simulink model "controlScheme_rt"  (R2017a)
settings: Solver=ode4  StartTime=0.0  StopTime=5000  FixedStep=1/30  RelTol=1e-3  EnableMultiTasking=on
PreLoadFcn:
  | target_ip_addr = '192.168.1.5';
  | target_user = 'root';
model workspace (MAT data in the model file):
  N_obj = Simulink.Parameter
  N_obj.Value = 1
  N_obj.DataType = 'auto'
  N_obj.Min = 0
  N_obj.Max = 4
  N_obj.Dimensions = [1 1]
  target_ip_addr = '147.32.86.138'
undefined symbols (not defined in the file): H, H_R
libraries: TB_blk_library x2
settings Model: SimulationMode=external  ExtModeTrigDuration=200000  Creator=krecmich  LastModifiedBy=gurtnmar
settings DataIOCC: LimitDataPoints=on  SaveFormat=Array
settings OptimizationCC: ExpressionDepthLimit=2147483647  LifeSpan=1
settings DebuggingCC: UnderspecifiedInitializationDetection=Classic  MergeDetectMultiDrivingBlocksExec=none  SolverPrmCheckMsg=warning  StateNameClashWarn=warning  SFUnexpectedBacktrackingDiag=warning  SFNoUnconditionalDefaultTransitionDiag=warning  SFExecutionAtInitializationDiag=none
settings HardwareCC: ProdBitPerLong=64  ProdLargestAtomicFloat=None  ProdHWDeviceType=Intel->x86-64
settings ModelReferenceCC: PropagateSignalLabelsOutOfModel=off
settings SFSimCC: MATLABDynamicMemAlloc=off
settings RTWCC: SystemTargetFile=ert_linux.tlc  MakeCommand="make_rtw OPT_OPTS=\"-O2 -ggdb -Wall\" CC=aarch64-linux-gnu-gcc CPP=aarch64-linux-gnu-gcc"  TemplateMakefile=ert_linux.tmf  Description=Linux Embedded Coder
settings CodeAppCC: IgnoreCustomStorageClasses=off  CustomSymbolStrType=$N$R$M  InternalIdentifier=Classic
settings STFCustomTargetCC: TargetLangStandard=C99 (ISO)  ModelReferenceCompliant=off  CombineOutputUpdateFcns=on  ERTCustomFileBanners=on  RemoveResetFunc=on  MATLABClassNameForMDSCustomization=Simulink.SoftwareTarget.ERTCustomization  GRTInterface=off  SystemTargetFile=ert_linux.tlc
settings ERTTargetCC: TargetLangStandard=C99 (ISO)  MultiwordLength=2048  ModelReferenceCompliant=off  ParMdlRefBuildCompliant=off  CompOptLevelCompliant=off  ConcurrentExecutionCompliant=off  ERTFirstTimeCompliant=off  SupportContinuousTime=on  SupportNonInlinedSFcns=on  ModelStepFunctionPrototypeControlCompliant=off  CPPClassGenCompliant=off  UseToolchainInfoCompliant=off  ExtMode=on  ExtModeMexArgs='147.32.86.138'  ERTCustomFileTemplate=ert_linux_file_process.tlc  ConvertIfToSwitch=off  SuppressUnreachableDefaultCases=off
settings ConfigComp: CovMetricSettings=dw  CovHtmlReporting=on  CovSaveCumulativeToWorkspaceVar=on  CovSaveSingleToWorkspaceVar=on  CovExternalEMLEnable=off

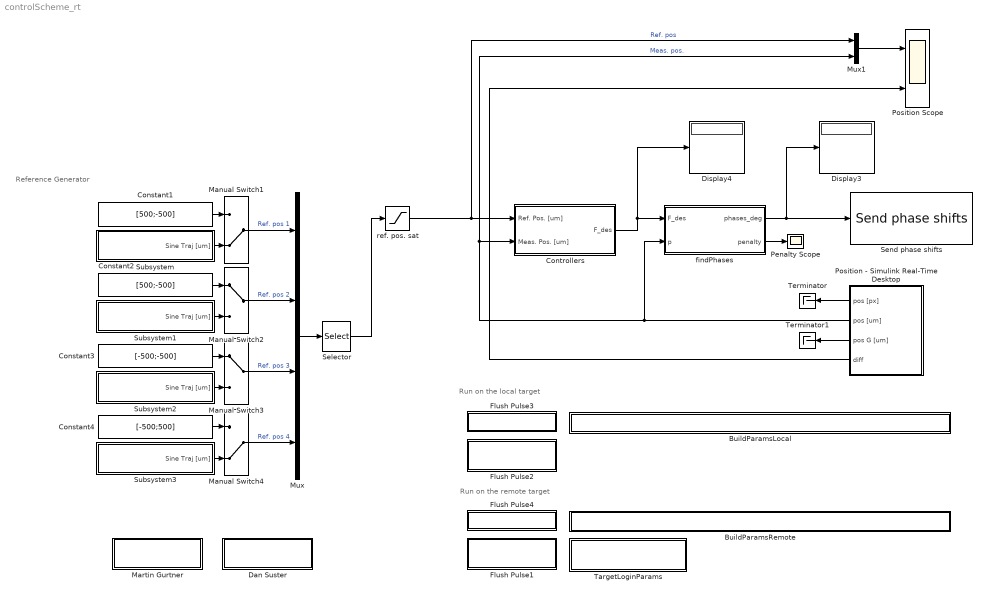
== system controlScheme_rt ==
  note: Reference Generator
  note: Run on the remote target
  note: Run on the local target
  BuildParamsLocal : Subsystem  mask{make_command='make_rtw OPT_OPTS="-O2 -ggdb -Wall" CC=gcc'}
      mask prompts: make_command "MakeCommand"
      mask Display: disp(get_param(gcb, 'make_command'));
  BuildParamsRemote : Subsystem  mask{make_command='make_rtw OPT_OPTS="-O2 -ggdb -Wall" CC=aarch64-linux-gnu-gcc CPP=aarch64-linux-gnu-gcc'}
      mask prompts: make_command "MakeCommand"
      mask Display: disp(get_param(gcb, 'make_command'));
  Constant1 : Constant  Value=[500;-500]
  Constant2 : Constant  Value=[500;-500]
  Constant3 : Constant  Value=[-500;-500]
  Constant4 : Constant  Value=[-500;500]
  Controllers : Subsystem  mask{P_const=300e-14, F_max=30e-11}
      mask prompts: P_const "P constant"; F_max "F max"
  Dan Suster : Subsystem
      settings: OpenFcn=|
      | wrkspc = get_param('controlScheme_rt', 'modelworkspace')
      | N_obj_sp = getVariable(wrkspc, 'N_obj')
      | N_obj = N_obj_sp.Value;
      | ip_addr = getVariable(wrkspc, 'target_ip_addr');
      | 
      | tb = twinbeam(ip_addr, 30000)
      | img_G = tb.get('backpropagated');
      | img_R = tb.get('backpropagated_r');
      | delete(tb);
      | %%
      | fig = figure(25);
      | imshow(img_G);
      | [x, y] = ginput(N_obj);
      | positions = [y, x];
      | positions_G = [positions(:,2)'; positions(:,1)'];
      | 
      | imshow(img_R);
      | [x, y] = ginput(N_obj);
      | positions = [y, x];
      | positions_R = [positions(:,2)'; positions(:,1)'];
      | 
      | close(fig);
      | %%
      | message = [uint8('t'), uint8('i'), typecast(uint16(numel(positions_G)/2),'uint8'), typecast(uint16(numel(positions_R)/2),'uint8'), typecast(uint16(positions_G(:)'),'uint8'), typecast(uint16(positions_R(:)'),'uint8')];
      | %%
      | conn = tcpclient('147.32.86.138', 30003, 'ConnectTimeout', 5);
      | write(conn, message);
      | clear conn;
      mask Display: disp('(Re)Initialize\ntracker')
  Display3 : Display
  Display4 : Display
  Flush Pulse1 : Subsystem
      settings: OpenFcn=|
      | % get the login credentials from the TargetLoginParams block
      | trgt_ip = eval(get_param(strcat(gcs, '/TargetLoginParams'), 'trgt_ip_addr'));
      | trgt_user = eval(get_param(strcat(gcs, '/TargetLoginParams'), 'trgt_username'));
      | 
      | % Set the IP address of the target
      | set_param(getActiveConfigSet(gcs), 'ExtModeMexArgs', sprintf('''%s''', trgt_ip));
      | 
      | system(['./run_model.sh ', get_param(bdroot(gcbh),'name'),' ',trgt_ip,' ',trgt_user]);
      mask Display: disp('Deploy and\nwait for connection')
  Flush Pulse2 : Subsystem
      settings: OpenFcn=|
      | configSet = getActiveConfigSet(gcs);
      | % Set the make command params
      | set_param( configSet, 'MakeCommand', '''make_rtw OPT_OPTS="-O2 -ggdb -Wall" CC=gcc''')
      | 
      | % Set the IP address of the target to the localhost
      | set_param(getActiveConfigSet(gcs), 'ExtModeMexArgs', '''127.0.0.1''')
      | 
      | system(['./run_model.sh ', get_param(bdroot(gcbh),'name')]);
      mask Display: disp('Deploy and\nwait for connection')
  Flush Pulse3 : Subsystem
      settings: OpenFcn=|
      | configSet = getActiveConfigSet(gcs);
      | % Set the make command params
      | set_param( configSet, 'MakeCommand', eval(get_param(strcat(gcs, '/BuildParamsLocal'), 'make_command')))
      | 
      | % Build the model
      | rtwbuild(gcs);
      mask Display: disp('Build')
  Flush Pulse4 : Subsystem
      settings: OpenFcn=|
      | configSet = getActiveConfigSet(gcs);
      | % Set the make command params
      | set_param( configSet, 'MakeCommand', eval(get_param(strcat(gcs, '/BuildParamsRemote'), 'make_command')))
      | 
      | % Build the model
      | rtwbuild(gcs);
      mask Display: disp('Build')
  Manual Switch1 : ManualSwitch  CurrentSetting=0
  Manual Switch2 : ManualSwitch
  Manual Switch3 : ManualSwitch
  Manual Switch4 : ManualSwitch  CurrentSetting=0
  Martin Gurtner : Subsystem
      settings: OpenFcn=|
      | wrkspc = get_param('controlScheme_rt', 'modelworkspace')
      | N_obj_sp = getVariable(wrkspc, 'N_obj')
      | N_obj = N_obj_sp.Value;
      | ip_addr = getVariable(wrkspc, 'target_ip_addr');
      | 
      | tb = twinbeam(ip_addr, 30000)
      | tb.tracker_init(N_obj);
      | clear conn;
      | delete(tb);
      mask Display: disp('(Re)Initialize\ntracker')
  Mux : Mux
  Mux1 : Mux  Inputs=2
  Penalty Scope : Scope
  Position - Simulink Real-Time Desktop : Subsystem  VariantControl=(default)
  Position Scope : Scope  NumInputPorts=2
  Selector : Selector  InputPortWidth=8  IndexOptions=Index vector (dialog)  Indices=[1:2*N_obj]  OutputSizes=1
  Send phase shifts : TB_blk_library/Send phase shifts  Ts=1/30  ip_addr=target_ip_addr  tcp_port=30001
  Subsystem : Subsystem  mask{xAmpl=400, xFreq=2*pi/50, xOff=0, yAmpl=400, yFreq=2*pi/50, yOff=pi/2}
      mask prompts: xAmpl "Amplitude"; xFreq "Frequency"; xOff "Phase Offset"; yAmpl "Amplitude"; yFreq "Frequency"; yOff "Phase Offset"
      mask DialogControl Container3 Prompt: Sine Trajectory Generator
      mask Display:
      | xAmpl = get_param(gcb, 'xAmpl');
      | xFreq = get_param(gcb, 'xFreq');
      | xOff = get_param(gcb, 'xOff');
      | yAmpl = get_param(gcb, 'yAmpl');
      | yFreq = get_param(gcb, 'yFreq');
      | yOff = get_param(gcb, 'yOff');
      | 
      | fprintf('x:%s sin(%s*t + %s)\ny:%s sin(%s*t + %s)', xAmpl, xFreq, xOff, yAmpl, yFreq, yOff)
  Subsystem1 : Subsystem  mask{xAmpl=300, xFreq=2*pi/40, xOff=pi/2, yAmpl=300, yFreq=2*pi/40, yOff=pi}
      mask prompts: xAmpl "Amplitude"; xFreq "Frequency"; xOff "Phase Offset"; yAmpl "Amplitude"; yFreq "Frequency"; yOff "Phase Offset"
      mask DialogControl Container3 Prompt: Sine Trajectory Generator
      mask Display:
      | xAmpl = get_param(gcb, 'xAmpl');
      | xFreq = get_param(gcb, 'xFreq');
      | xOff = get_param(gcb, 'xOff');
      | yAmpl = get_param(gcb, 'yAmpl');
      | yFreq = get_param(gcb, 'yFreq');
      | yOff = get_param(gcb, 'yOff');
      | 
      | fprintf('x:%s sin(%s*t + %s)\ny:%s sin(%s*t + %s)', xAmpl, xFreq, xOff, yAmpl, yFreq, yOff)
  Subsystem2 : Subsystem  mask{xAmpl=400, xFreq=2*pi/40, xOff=pi, yAmpl=400, yFreq=2*pi/40, yOff=3*pi/2}
      mask prompts: xAmpl "Amplitude"; xFreq "Frequency"; xOff "Phase Offset"; yAmpl "Amplitude"; yFreq "Frequency"; yOff "Phase Offset"
      mask DialogControl Container3 Prompt: Sine Trajectory Generator
      mask Display:
      | xAmpl = get_param(gcb, 'xAmpl');
      | xFreq = get_param(gcb, 'xFreq');
      | xOff = get_param(gcb, 'xOff');
      | yAmpl = get_param(gcb, 'yAmpl');
      | yFreq = get_param(gcb, 'yFreq');
      | yOff = get_param(gcb, 'yOff');
      | 
      | fprintf('x:%s sin(%s*t + %s)\ny:%s sin(%s*t + %s)', xAmpl, xFreq, xOff, yAmpl, yFreq, yOff)
  Subsystem3 : Subsystem  mask{xAmpl=400, xFreq=2*pi/40, xOff=3*pi/2, yAmpl=400, yFreq=2*pi/40, yOff=2*pi}
      mask prompts: xAmpl "Amplitude"; xFreq "Frequency"; xOff "Phase Offset"; yAmpl "Amplitude"; yFreq "Frequency"; yOff "Phase Offset"
      mask DialogControl Container3 Prompt: Sine Trajectory Generator
      mask Display:
      | xAmpl = get_param(gcb, 'xAmpl');
      | xFreq = get_param(gcb, 'xFreq');
      | xOff = get_param(gcb, 'xOff');
      | yAmpl = get_param(gcb, 'yAmpl');
      | yFreq = get_param(gcb, 'yFreq');
      | yOff = get_param(gcb, 'yOff');
      | 
      | fprintf('x:%s sin(%s*t + %s)\ny:%s sin(%s*t + %s)', xAmpl, xFreq, xOff, yAmpl, yFreq, yOff)
  TargetLoginParams : Subsystem  mask{trgt_ip_addr='147.32.86.138', trgt_username='nvidia'}
      mask prompts: trgt_ip_addr "Target IP address"; trgt_username "Target username"
      mask Display:
      | ip_addr = get_param(gcb, 'trgt_ip_addr');
      | user = get_param(gcb, 'trgt_username');
      | 
      | fprintf('IP addr:\t %s\n User:\t %s ', ip_addr, user);
  Terminator : Terminator
  Terminator1 : Terminator
  findPhases : MATLAB Function  TreatAsAtomicUnit=on
  ref. pos. sat : Saturate  UpperLimit=600  LowerLimit=-600
  wires:
  findPhases/2(penalty) -> Penalty Scope/1
  Position - Simulink Real-Time Desktop/2(pos [um]) -> findPhases/2(p), Controllers/2(Meas. Pos. [um]), Mux1/2  "Meas. pos."
  Controllers/1(F_des) -> findPhases/1(F_des), Display4/1
  findPhases/1(phases_deg) -> Send phase shifts/1, Display3/1
  Position - Simulink Real-Time Desktop/1(pos [px]) -> Terminator/1
  ref. pos. sat/1 -> Mux1/1, Controllers/1(Ref. Pos. [um])  "Ref. pos"
  Mux/1 -> Selector/1
  Position - Simulink Real-Time Desktop/3(pos G [um]) -> Terminator1/1
  Constant1/1 -> Manual Switch1/1
  Subsystem/1(Sine Traj [um]) -> Manual Switch1/2
  Subsystem1/1(Sine Traj [um]) -> Manual Switch2/2
  Constant2/1 -> Manual Switch2/1
  Constant3/1 -> Manual Switch3/1
  Subsystem2/1(Sine Traj [um]) -> Manual Switch3/2
  Subsystem3/1(Sine Traj [um]) -> Manual Switch4/2
  Constant4/1 -> Manual Switch4/1
  Manual Switch1/1 -> Mux/1  "Ref. pos 1"
  Manual Switch2/1 -> Mux/2  "Ref. pos 2"
  Manual Switch3/1 -> Mux/3  "Ref. pos 3"
  Manual Switch4/1 -> Mux/4  "Ref. pos 4"
  Selector/1 -> ref. pos. sat/1
  Mux1/1 -> Position Scope/1
  Position - Simulink Real-Time Desktop/4(diff) -> Position Scope/2

== system controlScheme_rt/BuildParamsLocal ==

== system controlScheme_rt/BuildParamsRemote ==

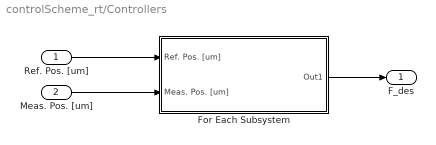
== system controlScheme_rt/Controllers ==
  Ref. Pos. [um] : Inport
  Meas. Pos. [um] : Inport  Port=2
  For Each Subsystem : Subsystem  TreatAsAtomicUnit=on
  F_des : Outport
  wires:
  Ref. Pos. [um]/1 -> For Each Subsystem/1(Ref. Pos. [um])
  For Each Subsystem/1(Out1) -> F_des/1
  Meas. Pos. [um]/1 -> For Each Subsystem/2(Meas. Pos. [um])

== system controlScheme_rt/Dan Suster ==

== system controlScheme_rt/Flush Pulse1 ==

== system controlScheme_rt/Flush Pulse2 ==

== system controlScheme_rt/Flush Pulse3 ==

== system controlScheme_rt/Flush Pulse4 ==

== system controlScheme_rt/Martin Gurtner ==

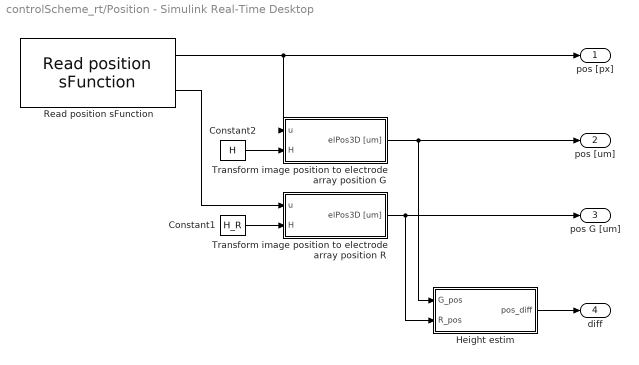
== system controlScheme_rt/Position - Simulink Real-Time Desktop ==
  Constant1 : Constant  Value=H_R
  Constant2 : Constant  Value=H
  Height estim : Subsystem  TreatAsAtomicUnit=on
  Read position sFunction : TB_blk_library/Read position sFunction  Ts=1/30  ip_addr=target_ip_addr  tcp_port=30002  N_objs=N_obj  track_in_RG=on
  Transform image position to electrode array position G : Subsystem  TreatAsAtomicUnit=on
  Transform image position to electrode array position R : Subsystem  TreatAsAtomicUnit=on
  pos [px] : Outport
  pos [um] : Outport  Port=2  Unit=um
  pos G [um] : Outport  Port=3  Unit=um
  diff : Outport  Port=4
  wires:
  Transform image position to electrode array position G/1(elPos3D [um]) -> pos [um]/1, Height estim/1(G_pos)
  Constant2/1 -> Transform image position to electrode array position G/2(H)
  Read position sFunction/1 -> pos [px]/1, Transform image position to electrode array position G/1(u)
  Height estim/1(pos_diff) -> diff/1
  Constant1/1 -> Transform image position to electrode array position R/2(H)
  Read position sFunction/2 -> Transform image position to electrode array position R/1(u)
  Transform image position to electrode array position R/1(elPos3D [um]) -> pos G [um]/1, Height estim/2(R_pos)

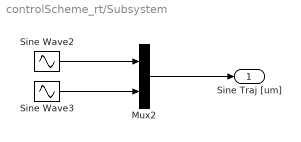
== system controlScheme_rt/Subsystem ==
  Mux2 : Mux  Inputs=2
  Sine Wave2 : Sin  Amplitude=xAmpl  Frequency=xFreq  Phase=xOff  SampleTime=0
  Sine Wave3 : Sin  Amplitude=yAmpl  Frequency=yFreq  Phase=yOff  SampleTime=0
  Sine Traj [um] : Outport
  wires:
  Mux2/1 -> Sine Traj [um]/1
  Sine Wave3/1 -> Mux2/2
  Sine Wave2/1 -> Mux2/1

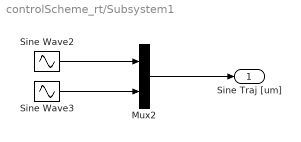
== system controlScheme_rt/Subsystem1 ==
  Mux2 : Mux  Inputs=2
  Sine Wave2 : Sin  Amplitude=xAmpl  Frequency=xFreq  Phase=xOff  SampleTime=0
  Sine Wave3 : Sin  Amplitude=yAmpl  Frequency=yFreq  Phase=yOff  SampleTime=0
  Sine Traj [um] : Outport
  wires:
  Sine Wave2/1 -> Mux2/1
  Sine Wave3/1 -> Mux2/2
  Mux2/1 -> Sine Traj [um]/1

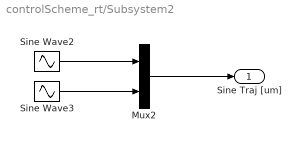
== system controlScheme_rt/Subsystem2 ==
  Mux2 : Mux  Inputs=2
  Sine Wave2 : Sin  Amplitude=xAmpl  Frequency=xFreq  Phase=xOff  SampleTime=0
  Sine Wave3 : Sin  Amplitude=yAmpl  Frequency=yFreq  Phase=yOff  SampleTime=0
  Sine Traj [um] : Outport
  wires:
  Mux2/1 -> Sine Traj [um]/1
  Sine Wave3/1 -> Mux2/2
  Sine Wave2/1 -> Mux2/1

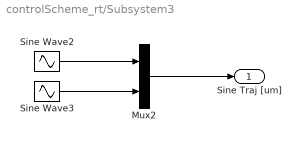
== system controlScheme_rt/Subsystem3 ==
  Mux2 : Mux  Inputs=2
  Sine Wave2 : Sin  Amplitude=xAmpl  Frequency=xFreq  Phase=xOff  SampleTime=0
  Sine Wave3 : Sin  Amplitude=yAmpl  Frequency=yFreq  Phase=yOff  SampleTime=0
  Sine Traj [um] : Outport
  wires:
  Sine Wave2/1 -> Mux2/1
  Sine Wave3/1 -> Mux2/2
  Mux2/1 -> Sine Traj [um]/1

== system controlScheme_rt/TargetLoginParams ==

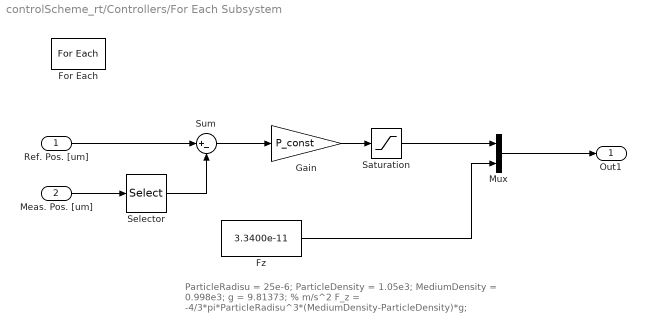
== system controlScheme_rt/Controllers/For Each Subsystem ==
  note: ParticleRadisu = 25e-6;
      | ParticleDensity = 1.05e3;
      | MediumDensity = 0.998e3;
      | g = 9.81373; % m/s^2
      | F_z = -4/3*pi*ParticleRadisu^3*(MediumDensity-ParticleDensity)*g;
  Ref. Pos. [um] : Inport  Partition=on  PartitionDimension=1  PartitionWidth=2
  Meas. Pos. [um] : Inport  Port=2  Partition=on  PartitionDimension=1  PartitionWidth=3
  For Each : ForEach  DisableCoverage=on
  Fz : Constant  Value=3.3400e-11
  Gain : Gain  Gain=P_const
  Mux : Mux  Inputs=2
  Saturation : Saturate  UpperLimit=F_max  LowerLimit=-F_max
  Selector : Selector  InputPortWidth=3  IndexOptions=Index vector (dialog)  Indices=[1 2]  OutputSizes=1
  Sum : Sum  Inputs=|+-
  Out1 : Outport  ConcatenationDimension=1
  wires:
  Gain/1 -> Saturation/1
  Mux/1 -> Out1/1
  Saturation/1 -> Mux/1
  Fz/1 -> Mux/2
  Meas. Pos. [um]/1 -> Selector/1
  Sum/1 -> Gain/1
  Selector/1 -> Sum/2
  Ref. Pos. [um]/1 -> Sum/1

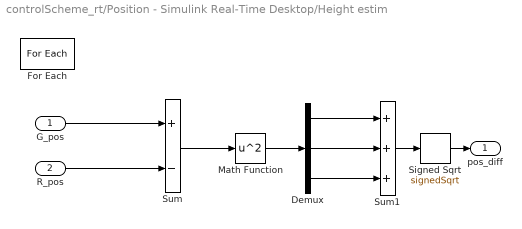
== system controlScheme_rt/Position - Simulink Real-Time Desktop/Height estim ==
  G_pos : Inport  Partition=on  PartitionDimension=1  PartitionWidth=3
  R_pos : Inport  Port=2  Partition=on  PartitionDimension=1  PartitionWidth=3
  Demux : Demux  Outputs=3
  For Each : ForEach  DisableCoverage=on
  Math Function : Math  Operator=square  SaturateOnIntegerOverflow=on
  Signed Sqrt : Sqrt  Operator=signedSqrt  SaturateOnIntegerOverflow=on
  Sum : Sum  Inputs=+-
  Sum1 : Sum  Inputs=+++
  pos_diff : Outport  ConcatenationDimension=1
  wires:
  G_pos/1 -> Sum/1
  R_pos/1 -> Sum/2
  Sum/1 -> Math Function/1
  Math Function/1 -> Demux/1
  Demux/1 -> Sum1/1
  Demux/2 -> Sum1/2
  Sum1/1 -> Signed Sqrt/1
  Demux/3 -> Sum1/3
  Signed Sqrt/1 -> pos_diff/1

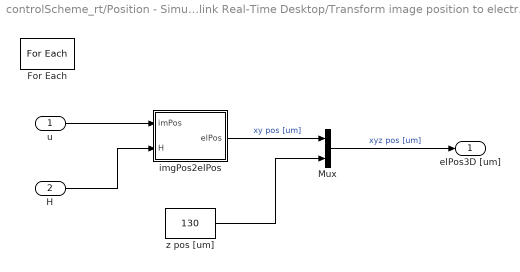
== system controlScheme_rt/Position - Simulink Real-Time Desktop/Transform image position to electrode array position G ==
  u : Inport  Partition=on  PartitionDimension=1  PartitionWidth=2
  H : Inport  Port=2
  For Each : ForEach  DisableCoverage=on
  Mux : Mux  Inputs=2
  imgPos2elPos : MATLAB Function  TreatAsAtomicUnit=on
  z pos [um] : Constant  Value=130
  elPos3D [um] : Outport  ConcatenationDimension=1
  wires:
  H/1 -> imgPos2elPos/2(H)
  u/1 -> imgPos2elPos/1(imPos)
  imgPos2elPos/1(elPos) -> Mux/1  "xy pos [um]"
  Mux/1 -> elPos3D [um]/1  "xyz pos [um]"
  z pos [um]/1 -> Mux/2

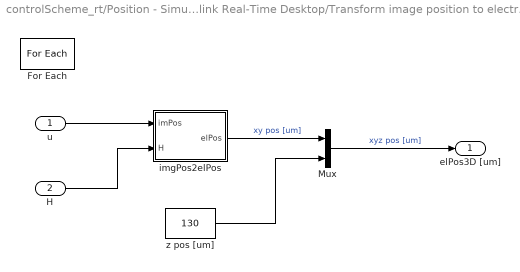
== system controlScheme_rt/Position - Simulink Real-Time Desktop/Transform image position to electrode array position R ==
  u : Inport  Partition=on  PartitionDimension=1  PartitionWidth=2
  H : Inport  Port=2
  For Each : ForEach  DisableCoverage=on
  Mux : Mux  Inputs=2
  imgPos2elPos : MATLAB Function  TreatAsAtomicUnit=on
  z pos [um] : Constant  Value=130
  elPos3D [um] : Outport  ConcatenationDimension=1
  wires:
  z pos [um]/1 -> Mux/2
  Mux/1 -> elPos3D [um]/1  "xyz pos [um]"
  imgPos2elPos/1(elPos) -> Mux/1  "xy pos [um]"
  u/1 -> imgPos2elPos/1(imPos)
  H/1 -> imgPos2elPos/2(H)

== matlab function controlScheme_rt/Position - Simulink Real-Time Desktop/Transform image position to electrode array position G/imgPos2elPos ==
  data: imPos input; elPos output; H input
function elPos = fcn(imPos, H)
tmp = H*[double(imPos(2));double(imPos(1));1];
elPos = [tmp(1)/tmp(3); tmp(2)/tmp(3)];

== matlab function controlScheme_rt/Position - Simulink Real-Time Desktop/Transform image position to electrode array position R/imgPos2elPos ==
  data: imPos input; elPos output; H input
function elPos = fcn(imPos, H)
tmp = H*[double(imPos(2));double(imPos(1));1];
elPos = [tmp(1)/tmp(3); tmp(2)/tmp(3)];

== matlab function controlScheme_rt/findPhases ==
  data: F_des input; p input; phases_deg output; penalty output
function [phases_deg, penalty] = fcn(F_des, p)
[phases_rad, penalty] = findPhasesFoGivenF(p*1e-6, F_des);
phases_deg_tmp = rad2deg(phases_rad);
phases_deg = uint16(round(mod(phases_deg_tmp, 360)));
